simulink model "IEEE_9bus_new_wow_mach_9"  (R2013a)
settings: Solver=ode8  StartTime=0.0  StopTime=3  RelTol=1e-4
PreLoadFcn:
  | ct = 1.083
undefined symbols (not defined in the file): D1, Delta
libraries: powerlib x37, jailib x3, sps_avr x3
settings Model: Creator=jp536285  LastModifiedBy=ChakZ
settings DataIOCC: LimitDataPoints=off  SaveOutput=off  SaveTime=off
settings DebuggingCC: UnconnectedInputMsg=none  UnconnectedOutputMsg=none  UnconnectedLineMsg=none

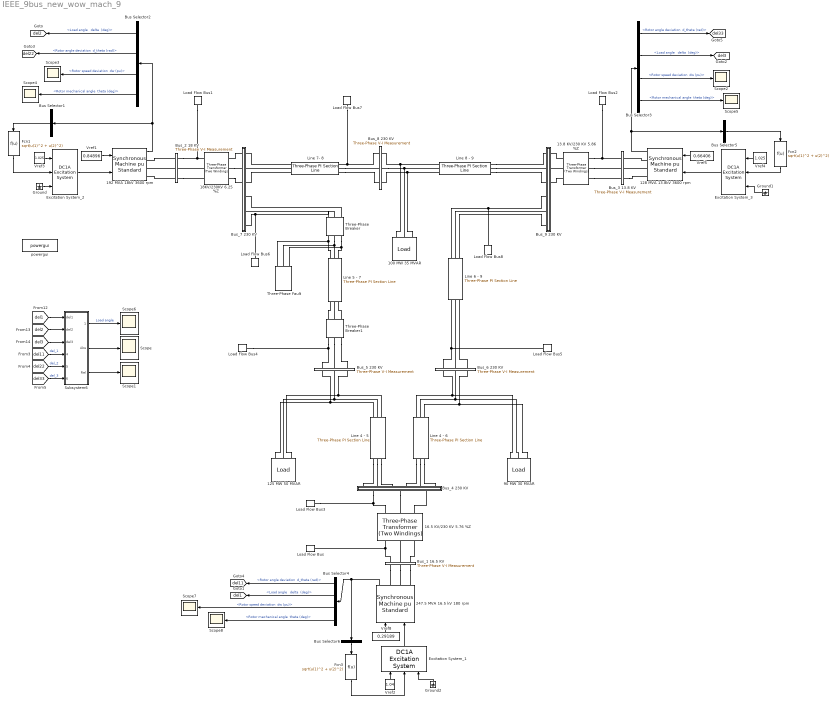
== system IEEE_9bus_new_wow_mach_9 ==
  " Line 4 - 6" : powerlib/Elements/Three-Phase PI Section Line  LConnTagsString=a|b|c  RConnTagsString=A|B|C  Frequency=60  Resistances=[ 0.08993 0.224825]  Inductances="[ 1.29e-3  3.22e-3]"  Capacitances=[7.922e-9 4.74e-9]  Length=100  mask(Three-Phase PI Section Line){}
      mask Display:
      | % This is a new mask on top of the base mask.
      | % Use "View base mask" link below to see the base mask.
      | patch([0.0 0.0 1 1 0.0 0.0 ],[0.4 0.7 0.7 0.4 0.4 0.7],[0 0 1]);
      | patch([0.4 0.4 0.42 0.42],[0.4 0.75 0.75 0.4],[1 0 0]);
      | patch([0.38 0.38 0.57 0.57],[0.7 0.75 0.75 0.7],[1 0 0]);
      | patch([0.53 0.53 0.55 0.55],[0.4 0.75 0.75 0.4],[1 0 0]);
  " Line 6 - 9" : powerlib/Elements/Three-Phase PI Section Line  LConnTagsString=a|b|c  RConnTagsString=A|B|C  Frequency=60  Resistances=[ 0.20631 0.5157]  Inductances="[ 2.38e-3  6.09e-3]"  Capacitances=[17.95e-9 10.55e-9]  Length=100  mask(Three-Phase PI Section Line){}
      mask Display:
      | % This is a new mask on top of the base mask.
      | % Use "View base mask" link below to see the base mask.
      | patch([0.0 0.0 1 1 0.0 0.0 ],[0.4 0.7 0.7 0.4 0.4 0.7],[0 0 1]);
      | patch([0.4 0.4 0.42 0.42],[0.4 0.75 0.75 0.4],[1 0 0]);
      | patch([0.38 0.38 0.57 0.57],[0.7 0.75 0.75 0.7],[1 0 0]);
      | patch([0.53 0.53 0.55 0.55],[0.4 0.75 0.75 0.4],[1 0 0]);
  100 MW 35 MVAR : jailib/Load  SystemSampleTime=-1
      link override Three-Phase Parallel RLC Load: NominalVoltage=(230000)*1.01602  ActivePower=100e6  InductivePower=35e6  LoadType=constant PQ
  125 MW 50 MVAR : jailib/Load  SystemSampleTime=-1
      link override Three-Phase Parallel RLC Load: NominalVoltage=(230000)*0.996183  ActivePower=125e6  InductivePower=50e6  LoadType=constant PQ
  128 MVA 13.8kV 3600 rpm : powerlib/Machines/Synchronous Machine pu Standard  PresetModel=No  MechanicalLoad=Mechanical power Pm  ShowDetailedParameters=on  RotorType=Round  NominalParameters="[ 128e6  13.8e3   60 ]"  Reactances1=[ 1.68, 0.23206, 0.19, 1.61, 0.23206, 0.19, 0.314]  Reactances2="[ 1.305, 0.296, 0.252, 0.474,  0.243,  0.18 ]"  dAxisTimeConstants=Open-circuit  qAxisTimeConstants=Open-circuit  TimeConstants1="[ 4.4849  0.0681  0.1  ]"  TimeConstants2=[ 5.89, 0.001,0.6, 0.001 ]  TimeConstants3="[  4.49  0.0681  0.0513  ]"  TimeConstants4=[ 8.0, 0.03, 0.3371, 0.0295 ]  TimeConstants5=[ 1.01, 0.053, 0.1 ]  TimeConstants6=[ 1.3201, 0.023, 1.0, 0.07 ]  TimeConstants7="[  1.01  0.053  0.051266  ]"  TimeConstants8=[ 1.3201, 0.0231, 0.3371, 0.0295 ]  StatorResistance=1e-7  Mechanical="[ 2.35  0 1 ]"  PolePairs=1  InitialConditions=[0 -36.0034 0.653061 0.653061 0.653061 11.785 -108.215 131.785 1.40359]  SetSaturation=off  Saturation=[0.6404,0.7127,0.8441,0.9214,0.9956,1.082,1.19,1.316,1.457;0.7,0.7698,0.8872,0.9466,0.9969,1.046,1.1,1.151,1.201]  Units=per unit standard parameters  LoadFlowParameters=[1 85000000 0 0 0]  TsPowergui=0  TsBlock=-1  IterativeModel=Trapezoidal non iterative  BusType=PV  Pref=85000000  Qref=0  Qmin=-Inf  Qmax=Inf  PLF=0  QLF=0
  13.8 KV/230 KV 5.86 %Z : powerlib/Elements/Three-Phase Transformer (Two Windings)  Winding1Connection=Delta (D1)  UNITS=pu  NominalPower=[ 100e6 , 60 ]  Winding1=[ 13.8e3 , 1e-6 , 0 ]  Winding2Connection=Yg  Winding2=[ 230e3 , 1e-6, 0.0586 ]  SetSaturation=off  Rm=500  Lm=500  Saturation=[ 0,0 ; 0.0024,1.2 ; 1.0,1.52 ]  Hysteresis=off  DataFile='hysteresis'  SetInitialFlux=off  InitialFluxes=[ 0.8 , -0.8 , 0.7 ]  Measurements=None  MoreParameters=off  BreakLoop=off  DataType=off  TransfoNumber=1
  "16.5 KV/230 KV 5.76 %Z     " : powerlib/Elements/Three-Phase Transformer (Two Windings)  Winding1Connection=Delta (D1)  UNITS=pu  NominalPower=[ 100e6 , 60 ]  Winding1=[ 16.5e3 , 1e-6, 0 ]  Winding2Connection=Yg  Winding2=[ 230e3 ,1e-6, 0.0576 ]  SetSaturation=off  Rm=500  Lm=500  Saturation=[ 0,0 ; 0.0024,1.2 ; 1.0,1.52 ]  Hysteresis=off  DataFile='hysteresis'  SetInitialFlux=off  InitialFluxes=[ 0.8 , -0.8 , 0.7 ]  Measurements=None  MoreParameters=off  BreakLoop=off  DataType=off  TransfoNumber=1
  18KV/230KV 6.25 %Z : powerlib/Elements/Three-Phase Transformer (Two Windings)  Winding1Connection=Delta (D1)  UNITS=pu  NominalPower=[ 100e6 , 60 ]  Winding1=[ 18e3 , 1e-6 , 0]  Winding2Connection=Yg  Winding2=[ 230e3 , 1e-6, 0.0625 ]  SetSaturation=off  Rm=500  Lm=500  Saturation=[ 0,0 ; 0.0024,1.2 ; 1.0,1.52 ]  Hysteresis=off  DataFile='hysteresis'  SetInitialFlux=off  InitialFluxes=[ 0.8 , -0.8 , 0.7 ]  Measurements=None  MoreParameters=off  BreakLoop=off  DataType=off  TransfoNumber=1
  192 MVA 18kV 3600 rpm : powerlib/Machines/Synchronous Machine pu Standard  PresetModel=No  MechanicalLoad=Mechanical power Pm  ShowDetailedParameters=on  RotorType=Round  NominalParameters="[ 192e6  18e3   60 ]"  Reactances1=[ 1.72, 0.23, 0.1728,1.65, 0.23, 0.1728, 0.4224 ]  Reactances2="[ 1.305, 0.296, 0.252, 0.474,  0.243,  0.18 ]"  dAxisTimeConstants=Open-circuit  qAxisTimeConstants=Open-circuit  TimeConstants1="[ 4.4849  0.0681  0.1  ]"  TimeConstants2=[ 6, 0.001, 0.53, 0.001]  TimeConstants3="[  4.49  0.0681  0.0513  ]"  TimeConstants4=[ 8.0, 0.03, 0.3371, 0.0295 ]  TimeConstants5=[ 1.01, 0.053, 0.1 ]  TimeConstants6=[ 1.3201, 0.023, 1.0, 0.07 ]  TimeConstants7="[  1.01  0.053  0.051266  ]"  TimeConstants8=[ 1.3201, 0.0231, 0.3371, 0.0295 ]  StatorResistance=1e-7  Mechanical="[ 3.33  0 1 ]"  PolePairs=1  InitialConditions=[0 -29.1799 0.828949 0.828949 0.828949 6.81655 -113.183 126.817 1.78946]  SetSaturation=off  Saturation=[0.6404,0.7127,0.8441,0.9214,0.9956,1.082,1.19,1.316,1.457;0.7,0.7698,0.8872,0.9466,0.9969,1.046,1.1,1.151,1.201]  Units=per unit standard parameters  LoadFlowParameters=[1 163000000 0 0 0]  TsPowergui=0  TsBlock=-1  IterativeModel=Trapezoidal non iterative  BusType=PV  Pref=163000000  Qref=0  Qmin=-Inf  Qmax=Inf  PLF=0  QLF=0
  247.5 MVA 16.5 kV 180 rpm : powerlib/Machines/Synchronous Machine pu Standard  PresetModel=No  MechanicalLoad=Mechanical power Pm  ShowDetailedParameters=on  RotorType=Salient-pole  NominalParameters="[ 247.5E6  16500   60 ]"  Reactances1=[ 31 32 33 34 35 36 37 ]  Reactances2=[ 0.361, 0.1504, 0.099, 0.2398, 0.099, 0.062 ]  dAxisTimeConstants=Open-circuit  qAxisTimeConstants=Open-circuit  TimeConstants1=[8.96 0.001 0.001]  TimeConstants2=[]  TimeConstants3=[]  TimeConstants4=[]  TimeConstants5=[ 1.01, 0.053, 0.31 ]  TimeConstants6=[]  TimeConstants7=[]  TimeConstants8=[]  StatorResistance=1e-7  Mechanical=[9.55 0 20]  PolePairs=20  InitialConditions=[0 -86.3839 0.299344 0.299344 0.299344 -20.3492 -140.349 99.6508 1.08182]  SetSaturation=off  Saturation=[0.6404,0.7127,0.8441,0.9214,0.9956,1.082,1.19,1.316,1.457;0.7,0.7698,0.8872,0.9466,0.9969,1.046,1.1,1.151,1.201]  Units=per unit standard parameters  LoadFlowParameters=[2 71000000 0 0]  TsPowergui=0  TsBlock=-1  IterativeModel=Trapezoidal non iterative  BusType=swing  Pref=150000000  Qref=0  Qmin=-Inf  Qmax=Inf  PLF=0  QLF=0
      settings: AttributesFormatString=\n\n
  90 MW 30 MVAR : jailib/Load  SystemSampleTime=-1
      link override Three-Phase Parallel RLC Load: NominalVoltage=(230000)*1.01315  ActivePower=90e6  InductivePower=30e6  LoadType=constant PQ
  Bus Selector1 : BusSelector  OutputSignals="dq0 components.Stator voltage  vq (pu),dq0 components.Stator voltage  vd (pu)"  OutputAsBus=on
  Bus Selector2 : BusSelector  OutputSignals="Load angle   delta  (deg),Mechanical.Rotor angle deviation  d_theta (rad),Mechanical.Rotor speed deviation  dw (pu),Mechanical.Rotor mechanical angle  theta (deg)"
  Bus Selector3 : BusSelector  OutputSignals="Mechanical.Rotor angle deviation  d_theta (rad),Load angle   delta  (deg),Mechanical.Rotor speed deviation  dw (pu),Mechanical.Rotor mechanical angle  theta (deg)"
  Bus Selector4 : BusSelector  OutputSignals="Mechanical.Rotor angle deviation  d_theta (rad),Load angle   delta  (deg),Mechanical.Rotor speed deviation  dw (pu),Mechanical.Rotor mechanical angle  theta (deg)"
  Bus Selector5 : BusSelector  OutputSignals="dq0 components.Stator voltage  vq (pu),dq0 components.Stator voltage  vd (pu)"  OutputAsBus=on
  Bus Selector6 : BusSelector  OutputSignals="dq0 components.Stator voltage  vq (pu),dq0 components.Stator voltage  vd (pu)"  OutputAsBus=on
  Bus_1 16.5 KV : powerlib/Measurements/Three-Phase V-I Measurement  VoltageMeasurement=phase-to-phase  SetLabelV=on  LabelV=Vabc_1  Vpu=on  VpuLL=off  CurrentMeasurement=yes  SetLabelI=on  LabelI=Iabc_1  Ipu=on  Pbase=100e6  Vbase=16.5e3  OutputType=Complex  PhasorSimulation=off  PSBequivalent=0
  Bus_2 18 KV : powerlib/Measurements/Three-Phase V-I Measurement  VoltageMeasurement=phase-to-phase  SetLabelV=on  LabelV=Vabc_2  Vpu=on  VpuLL=off  CurrentMeasurement=yes  SetLabelI=on  LabelI=Iabc_2  Ipu=on  Pbase=100e6  Vbase=18e3  OutputType=Complex  PhasorSimulation=off  PSBequivalent=0
  Bus_3 13.8 KV : powerlib/Measurements/Three-Phase V-I Measurement  VoltageMeasurement=phase-to-phase  SetLabelV=on  LabelV=Vabc_3  Vpu=on  VpuLL=off  CurrentMeasurement=yes  SetLabelI=on  LabelI=Iabc_3  Ipu=on  Pbase=100e6  Vbase=13.8e3  OutputType=Complex  PhasorSimulation=off  PSBequivalent=0
  Bus_4 230 KV : Subsystem
  Bus_5 230 KV : powerlib/Measurements/Three-Phase V-I Measurement  VoltageMeasurement=phase-to-ground  SetLabelV=on  LabelV=Vabc_5  Vpu=on  VpuLL=off  CurrentMeasurement=yes  SetLabelI=on  LabelI=Iabc_5  Ipu=on  Pbase=100e6  Vbase=230e3  OutputType=Complex  PhasorSimulation=off  PSBequivalent=0
  Bus_6 230 KV : powerlib/Measurements/Three-Phase V-I Measurement  VoltageMeasurement=phase-to-ground  SetLabelV=on  LabelV=Vabc_6  Vpu=on  VpuLL=off  CurrentMeasurement=yes  SetLabelI=on  LabelI=Iabc_6  Ipu=on  Pbase=100e6  Vbase=230e3  OutputType=Complex  PhasorSimulation=off  PSBequivalent=0
  Bus_7 230 KV : Subsystem
  Bus_8 230 KV : powerlib/Measurements/Three-Phase V-I Measurement  VoltageMeasurement=phase-to-ground  SetLabelV=on  LabelV=Vabc_8  Vpu=on  VpuLL=off  CurrentMeasurement=yes  SetLabelI=on  LabelI=Iabc_8  Ipu=on  Pbase=100e6  Vbase=230e3  OutputType=Complex  PhasorSimulation=off  PSBequivalent=0
  Bus_9 230 KV : Subsystem
  Excitation System_2 : sps_avr/DC1A Excitation System  Tr=20e-3  KaTa=[20 0.2]  VRminmax=[ -4 4]  KfTf=[0.063 0.35]  TbTc=[0 0]  KeTe=[1 0.314]  Efd12=[3.1 2.3]  SeEfd12=[0.483 0.1394]  v0=[1.025 1.7895]  TsBlock=0
  Excitation System_1 : sps_avr/DC1A Excitation System  Tr=20e-3  KaTa=[20 0.2]  VRminmax=[ -3 3]  KfTf=[0.063 0.35]  TbTc=[0 0]  KeTe=[1 0.314]  Efd12=[3.1 2.3]  SeEfd12=[0.483 0.1394]  v0=[1.04 1.0818]  TsBlock=0
  Excitation System_3 : sps_avr/DC1A Excitation System  Tr=20e-3  KaTa=[20 0.2]  VRminmax=[-4 4]  KfTf=[0.063 0.35]  TbTc=[0 0]  KeTe=[1 0.314]  Efd12=[3.1 2.3]  SeEfd12=[0.483 0.1394]  v0=[1.025 1.4036]  TsBlock=0
  Fcn1 : Fcn  Expr=sqrt(u(1)^2 + u(2)^2)
  Fcn2 : Fcn  Expr=sqrt(u(1)^2 + u(2)^2)
  Fcn3 : Fcn  Expr=sqrt(u(1)^2 + u(2)^2)
  Ground : Ground
  Ground1 : Ground
  Ground2 : Ground
  "Line 4 - 5 " : powerlib/Elements/Three-Phase PI Section Line  LConnTagsString=a|b|c  RConnTagsString=A|B|C  Frequency=60  Resistances=[ 0.0529 0.13225]  Inductances="[ 1.192e-3  2.38e-3]"  Capacitances=[8.82e-9 5.188e-9]  Length=100  mask(Three-Phase PI Section Line){}
      mask Display:
      | % This is a new mask on top of the base mask.
      | % Use "View base mask" link below to see the base mask.
      | patch([0.0 0.0 1 1 0.0 0.0 ],[0.4 0.7 0.7 0.4 0.4 0.7],[0 0 1]);
      | patch([0.4 0.4 0.42 0.42],[0.4 0.75 0.75 0.4],[1 0 0]);
      | patch([0.38 0.38 0.57 0.57],[0.7 0.75 0.75 0.7],[1 0 0]);
      | patch([0.53 0.53 0.55 0.55],[0.4 0.75 0.75 0.4],[1 0 0]);
  "Line 5 - 7 " : powerlib/Elements/Three-Phase PI Section Line  LConnTagsString=a|b|c  RConnTagsString=A|B|C  Frequency=60  Resistances=[ 0.16928 0.4232]  Inductances="[ 2.259e-3  5.64e-3]"  Capacitances=[15.34e-9 9.025e-9]  Length=100  mask(Three-Phase PI Section Line){}
      mask Display:
      | % This is a new mask on top of the base mask.
      | % Use "View base mask" link below to see the base mask.
      | patch([0.0 0.0 1 1 0.0 0.0 ],[0.4 0.7 0.7 0.4 0.4 0.7],[0 0 1]);
      | patch([0.4 0.4 0.42 0.42],[0.4 0.75 0.75 0.4],[1 0 0]);
      | patch([0.38 0.38 0.57 0.57],[0.7 0.75 0.75 0.7],[1 0 0]);
      | patch([0.53 0.53 0.55 0.55],[0.4 0.75 0.75 0.4],[1 0 0]);
  Line 7- 8 : powerlib/Elements/Three-Phase PI Section Line  LConnTagsString=a|b|c  RConnTagsString=A|B|C  Frequency=60  Resistances=[0.044965 0.11241]  Inductances="[ 1.01e-3  2.02e-3]"  Capacitances=[7.471e-9 4.394e-9]  Length=100  mask(Three-Phase PI Section Line){}
      mask Display:
      | % This is a new mask on top of the base mask.
      | % Use "View base mask" link below to see the base mask.
      | patch([0.0 0.0 1 1 0.0 0.0 ],[0.4 0.7 0.7 0.4 0.4 0.7],[0 0 1]);
      | patch([0.4 0.4 0.42 0.42],[0.4 0.75 0.75 0.4],[1 0 0]);
      | patch([0.38 0.38 0.57 0.57],[0.7 0.75 0.75 0.7],[1 0 0]);
      | patch([0.53 0.53 0.55 0.55],[0.4 0.75 0.75 0.4],[1 0 0]);
  Line 8 - 9 : powerlib/Elements/Three-Phase PI Section Line  LConnTagsString=a|b|c  RConnTagsString=A|B|C  Frequency=60  Resistances=[ 0.062951 0.15737]  Inductances="[ 1.414e-3  3.53e-3]"  Capacitances=[10.47e-9 6.15e-9]  Length=100  mask(Three-Phase PI Section Line){}
      mask Display:
      | % This is a new mask on top of the base mask.
      | % Use "View base mask" link below to see the base mask.
      | patch([0.0 0.0 1 1 0.0 0.0 ],[0.4 0.7 0.7 0.4 0.4 0.7],[0 0 1]);
      | patch([0.4 0.4 0.42 0.42],[0.4 0.75 0.75 0.4],[1 0 0]);
      | patch([0.38 0.38 0.57 0.57],[0.7 0.75 0.75 0.7],[1 0 0]);
      | patch([0.53 0.53 0.55 0.55],[0.4 0.75 0.75 0.4],[1 0 0]);
  Load Flow Bus : powerlib/Measurements/Load Flow Bus  LConnTagsString=a  ID=BUS_1  Vbase=16.5e3  Vref=1.04  Vangle=0  VLF=1.04  angleLF=0
      settings: AttributesFormatString=%<ID>\n%<Vbase>V\n%<VLF>pu\n%<angleLF>deg.
  Load Flow Bus1 : powerlib/Measurements/Load Flow Bus  LConnTagsString=a  ID=BUS_2  Vbase=18e3  Vref=1.025  Vangle=0  VLF=1.025  angleLF=9.166
      settings: AttributesFormatString=%<ID>\n%<Vbase>V\n%<VLF>pu\n%<angleLF>deg.
  Load Flow Bus2 : powerlib/Measurements/Load Flow Bus  LConnTagsString=a  ID=BUS_3  Vbase=13.8e3  Vref=1.025  Vangle=0  VLF=1.025  angleLF=4.553
      settings: AttributesFormatString=%<ID>\n%<Vbase>V\n%<VLF>pu\n%<angleLF>deg.
  Load Flow Bus3 : powerlib/Measurements/Load Flow Bus  LConnTagsString=a  ID=BUS_4  Vbase=230e3  Vref=1  Vangle=0  VLF=1.026  angleLF=27.77
      settings: AttributesFormatString=%<ID>\n%<Vbase>V\n%<VLF>pu\n%<angleLF>deg.
  Load Flow Bus4 : powerlib/Measurements/Load Flow Bus  LConnTagsString=a  ID=BUS_5  Vbase=230e3  Vref=1  Vangle=0  VLF=0.9962  angleLF=25.99
      settings: AttributesFormatString=%<ID>\n%<Vbase>V\n%<VLF>pu\n%<angleLF>deg.
  Load Flow Bus5 : powerlib/Measurements/Load Flow Bus  LConnTagsString=a  ID=BUS_6  Vbase=230e3  Vref=1  Vangle=0  VLF=1.013  angleLF=26.3
      settings: AttributesFormatString=%<ID>\n%<Vbase>V\n%<VLF>pu\n%<angleLF>deg.
  Load Flow Bus6 : powerlib/Measurements/Load Flow Bus  LConnTagsString=a  ID=BUS_7  Vbase=230e3  Vref=1  Vangle=0  VLF=1.026  angleLF=33.61
      settings: AttributesFormatString=%<ID>\n%<Vbase>V\n%<VLF>pu\n%<angleLF>deg.
  Load Flow Bus7 : powerlib/Measurements/Load Flow Bus  LConnTagsString=a  ID=BUS_8  Vbase=230e3  Vref=1  Vangle=0  VLF=1.016  angleLF=30.63
      settings: AttributesFormatString=%<ID>\n%<Vbase>V\n%<VLF>pu\n%<angleLF>deg.
  Load Flow Bus8 : powerlib/Measurements/Load Flow Bus  LConnTagsString=a  ID=BUS_9  Vbase=230e3  Vref=1  Vangle=0  VLF=1.032  angleLF=31.86
      settings: AttributesFormatString=%<ID>\n%<Vbase>V\n%<VLF>pu\n%<angleLF>deg.
  Scope{,1..8} (9 alike) : Scope
      Scope settings: ShowLegends=on  YMin=-100  YMax=225
      Scope1 settings: ShowLegends=on  TimeRange=3.99997  YMin=51.5  YMax=59.5
      Scope2 settings: ShowLegends=on  YMin=-7.5  YMax=12.5  SaveName=ScopeData2
      Scope3 settings: ShowLegends=on  YMin=-7.5  YMax=12.5  SaveName=ScopeData3
      Scope4 settings: ShowLegends=on  YMin=-7.5  YMax=12.5  SaveName=ScopeData4
      Scope5 settings: ShowLegends=on  YMin=-7.5  YMax=12.5  SaveName=ScopeData5
      Scope6 settings: ShowLegends=on  YMin=-200  YMax=200  SaveName=ScopeData6
      Scope7 settings: ShowLegends=on  YMin=-7.5  YMax=12.5  SaveName=ScopeData7
      Scope8 settings: ShowLegends=on  YMin=-7.5  YMax=12.5  SaveName=ScopeData8
  Subsystem6 : Subsystem
  Three-Phase Breaker : powerlib/Elements/Three-Phase Breaker  InitialState=closed  SwitchA=on  SwitchB=on  SwitchC=on  SwitchTimes=[ct]  External=off  BreakerResistance=0.001  SnubberResistance=1e7  SnubberCapacitance=inf  Measurements=None
  Three-Phase Breaker1 : powerlib/Elements/Three-Phase Breaker  InitialState=closed  SwitchA=on  SwitchB=on  SwitchC=on  SwitchTimes=[ct]  External=off  BreakerResistance=0.001  SnubberResistance=1e7  SnubberCapacitance=inf  Measurements=None
  Three-Phase Fault : powerlib/Elements/Three-Phase Fault  FaultA=on  FaultB=on  FaultC=on  FaultResistance=0.001  GroundFault=on  GroundResistance=0.001  External=off  SwitchStatus=[1 0]  SwitchTimes=[ 1 ct]  InitialStates=[0 0 1]  SnubberResistance=1e6  SnubberCapacitance=inf  Measurements=None
  Vref1 : Constant  Value=0.84896
  Vref2 : Constant  Value=1.04
  Vref3 : Constant  Value=1.025
  Vref4 : Constant  Value=1.025
  Vref5 : Constant  Value=0.66406
  Vref8 : Constant  Value=0.29189
  powergui : powerlib/powergui  Priority=1  SimulationMode=Discrete  SolverType=Backward Euler  SampleTime=5e-5  frequency=60  SPID=off  DisableSnubberDevices=off  DisableRonSwitches=off  DisableVfSwitches=off  SwTol=0  Interpol=off  DisplayEquations=off  frequencyindice=60  Pbase=10e7  ErrMax=1e-05  Iterations=50  UnitsV=kV  UnitsW=MW  FunctionMessages=off  echomessages=off  HookPort=off  EnableUseOfTLC=off  x0status=blocks  RestoreLinks=warning  ResistiveCurrentMeasurement=off  Frange=[0:2:500]  Ylog=off  Xlog=on  ShowGrid=off  save=off  variable=ZData  ZoomFFT=off  StartTime=0.0  cycles=1  DisplayStyle=1  fundamental=60  FreqAxis=off  MaxFrequency=1000  frequencyindicesteady=1  RmsSteady=1  display=off  Ts=0  methode=off
  tag scope: del11=global, del1=global, del22=global, del2=global, del33=global, del3=global
  wires:
  Vref5/1 -> 128 MVA 13.8kV 3600 rpm/1
  Excitation System_3/1 -> 128 MVA 13.8kV 3600 rpm/2
  192 MVA 18kV 3600 rpm/1 -> Bus Selector2/1, Bus Selector1/1
  Bus Selector2/1 -> [del2]  "<Load angle   delta  (deg)>"
  Bus Selector3/2 -> [del3]  "<Load angle   delta  (deg)>"
  128 MVA 13.8kV 3600 rpm/1 -> Bus Selector3/1, Bus Selector5/1
  247.5 MVA 16.5 kV 180 rpm/1 -> Bus Selector4/1, Bus Selector6/1
  Vref8/1 -> 247.5 MVA 16.5 kV 180 rpm/1
  Excitation System_1/1 -> 247.5 MVA 16.5 kV 180 rpm/2
  Bus Selector4/2 -> [del1]  "<Load angle   delta  (deg)>"
  Vref3/1 -> Excitation System_2/1
  Ground/1 -> Excitation System_2/3
  Vref4/1 -> Excitation System_3/1
  Ground1/1 -> Excitation System_3/3
  Vref2/1 -> Excitation System_1/1
  Bus Selector2/2 -> [del22]  "<Rotor angle deviation  d_theta (rad)>"
  Bus Selector4/1 -> [del11]  "<Rotor angle deviation  d_theta (rad)>"
  Bus Selector3/1 -> [del33]  "<Rotor angle deviation  d_theta (rad)>"
  Bus Selector2/3 -> Scope3/1  "<Rotor speed deviation  dw (pu)>"
  Vref1/1 -> 192 MVA 18kV 3600 rpm/1
  [del1] -> Subsystem6/1(del1)
  [del2] -> Subsystem6/2(del2)
  [del3] -> Subsystem6/3(del3)
  Subsystem6/1(Load ang) -> Scope6/1  "Load angle"
  Bus Selector2/4 -> Scope4/1  "<Rotor mechanical angle  theta (deg)>"
  Bus Selector3/3 -> Scope2/1  "<Rotor speed deviation  dw (pu)>"
  Bus Selector3/4 -> Scope5/1  "<Rotor mechanical angle  theta (deg)>"
  Bus Selector4/3 -> Scope7/1  "<Rotor speed deviation  dw (pu)>"
  Bus Selector4/4 -> Scope8/1  "<Rotor mechanical angle  theta (deg)>"
  [del11] -> Subsystem6/4(del11)  "del_1"
  [del22] -> Subsystem6/5(del22)  "del_2"
  [del33] -> Subsystem6/6(del33)  "del_3"
  Subsystem6/2(Abs) -> Scope/1
  Subsystem6/3(Rel) -> Scope1/1
  Bus Selector1/1 -> Fcn1/1
  Fcn1/1 -> Excitation System_2/2
  Excitation System_2/1 -> 192 MVA 18kV 3600 rpm/2
  Bus Selector5/1 -> Fcn2/1
  Fcn2/1 -> Excitation System_3/2
  Ground2/1 -> Excitation System_1/3
  Bus Selector6/1 -> Fcn3/1
  Fcn3/1 -> Excitation System_1/2
  connections:
  Bus_2 18 KV/LConn2 -- 192 MVA 18kV 3600 rpm/RConn2
  18KV/230KV 6.25 %Z/LConn2 -- Bus_2 18 KV/RConn2
  18KV/230KV 6.25 %Z/RConn2 -- Bus_7 230 KV/LConn2
  Bus_2 18 KV/RConn1 -- Load Flow Bus1/LConn1 -- 18KV/230KV 6.25 %Z/LConn1
  Bus_2 18 KV/RConn3 -- 18KV/230KV 6.25 %Z/LConn3
  Bus_7 230 KV/LConn1 -- 18KV/230KV 6.25 %Z/RConn1
  18KV/230KV 6.25 %Z/RConn3 -- Bus_7 230 KV/LConn3
  13.8 KV/230 KV 5.86 %Z/LConn1 -- Bus_3 13.8 KV/LConn1 -- Load Flow Bus2/LConn1
  13.8 KV/230 KV 5.86 %Z/LConn2 -- Bus_3 13.8 KV/LConn2
  13.8 KV/230 KV 5.86 %Z/LConn3 -- Bus_3 13.8 KV/LConn3
  Bus_1 16.5 KV/RConn1 -- 247.5 MVA 16.5 kV 180 rpm/RConn1
  Bus_1 16.5 KV/RConn2 -- 247.5 MVA 16.5 kV 180 rpm/RConn2
  Bus_1 16.5 KV/RConn3 -- 247.5 MVA 16.5 kV 180 rpm/RConn3
  Bus_1 16.5 KV/LConn3 -- "16.5 KV/230 KV 5.76 %Z     "/LConn3
  Bus_1 16.5 KV/LConn2 -- "16.5 KV/230 KV 5.76 %Z     "/LConn2
  13.8 KV/230 KV 5.86 %Z/RConn1 -- Bus_9 230 KV/RConn1
  13.8 KV/230 KV 5.86 %Z/RConn2 -- Bus_9 230 KV/RConn2
  13.8 KV/230 KV 5.86 %Z/RConn3 -- Bus_9 230 KV/RConn3
  Bus_4 230 KV/LConn1 -- "16.5 KV/230 KV 5.76 %Z     "/RConn1 -- Load Flow Bus3/LConn1
  Bus_4 230 KV/LConn2 -- "16.5 KV/230 KV 5.76 %Z     "/RConn2
  Line 8 - 9/LConn1 -- Bus_8 230 KV/LConn1 -- 100 MW 35 MVAR/LConn1
  Line 8 - 9/LConn2 -- 100 MW 35 MVAR/LConn2 -- Bus_8 230 KV/LConn2
  Line 8 - 9/LConn3 -- 100 MW 35 MVAR/LConn3 -- Bus_8 230 KV/LConn3
  "16.5 KV/230 KV 5.76 %Z     "/RConn3 -- Bus_4 230 KV/LConn3
  "Line 4 - 5 "/LConn1 -- 125 MW 50 MVAR/LConn1 -- Bus_5 230 KV/RConn1
  "Line 4 - 5 "/LConn2 -- 125 MW 50 MVAR/LConn2 -- Bus_5 230 KV/RConn2
  "Line 4 - 5 "/LConn3 -- 125 MW 50 MVAR/LConn3 -- Bus_5 230 KV/RConn3
  " Line 4 - 6"/LConn1 -- 90 MW 30 MVAR/LConn1 -- Bus_6 230 KV/RConn1
  " Line 4 - 6"/LConn2 -- 90 MW 30 MVAR/LConn2 -- Bus_6 230 KV/RConn2
  " Line 4 - 6"/LConn3 -- 90 MW 30 MVAR/LConn3 -- Bus_6 230 KV/RConn3
  Line 7- 8/LConn1 -- Bus_7 230 KV/RConn1
  Line 7- 8/LConn2 -- Bus_7 230 KV/RConn2
  Bus_7 230 KV/RConn3 -- Line 7- 8/LConn3
  Bus_8 230 KV/RConn1 -- Line 7- 8/RConn1 -- Load Flow Bus7/LConn1
  Line 7- 8/RConn2 -- Bus_8 230 KV/RConn2
  Line 7- 8/RConn3 -- Bus_8 230 KV/RConn3
  Line 8 - 9/RConn2 -- Bus_9 230 KV/LConn2
  Line 8 - 9/RConn1 -- Bus_9 230 KV/LConn1
  Line 8 - 9/RConn3 -- Bus_9 230 KV/LConn3
  Bus_7 230 KV/RConn6 -- Three-Phase Breaker/LConn1 -- Load Flow Bus6/LConn1
  " Line 6 - 9"/RConn1 -- Load Flow Bus8/LConn1 -- Bus_9 230 KV/LConn4
  Bus_9 230 KV/LConn5 -- " Line 6 - 9"/RConn2
  Bus_6 230 KV/LConn1 -- " Line 6 - 9"/LConn1 -- Load Flow Bus5/LConn1
  Bus_6 230 KV/LConn2 -- " Line 6 - 9"/LConn2
  Bus_6 230 KV/LConn3 -- " Line 6 - 9"/LConn3
  " Line 6 - 9"/RConn3 -- Bus_9 230 KV/LConn6
  "Line 4 - 5 "/RConn2 -- Bus_4 230 KV/RConn2
  "Line 4 - 5 "/RConn1 -- Bus_4 230 KV/RConn1
  "Line 4 - 5 "/RConn3 -- Bus_4 230 KV/RConn3
  " Line 4 - 6"/RConn2 -- Bus_4 230 KV/RConn5
  " Line 4 - 6"/RConn1 -- Bus_4 230 KV/RConn4
  " Line 4 - 6"/RConn3 -- Bus_4 230 KV/RConn6
  128 MVA 13.8kV 3600 rpm/RConn1 -- Bus_3 13.8 KV/RConn1
  128 MVA 13.8kV 3600 rpm/RConn2 -- Bus_3 13.8 KV/RConn2
  Bus_3 13.8 KV/RConn3 -- 128 MVA 13.8kV 3600 rpm/RConn3
  Bus_2 18 KV/LConn3 -- 192 MVA 18kV 3600 rpm/RConn3
  Bus_2 18 KV/LConn1 -- 192 MVA 18kV 3600 rpm/RConn1
  Bus_1 16.5 KV/LConn1 -- Load Flow Bus/LConn1 -- "16.5 KV/230 KV 5.76 %Z     "/LConn1
  Three-Phase Breaker/RConn2 -- Three-Phase Fault/LConn2 -- "Line 5 - 7 "/LConn2
  Three-Phase Breaker/RConn1 -- Three-Phase Fault/LConn1 -- "Line 5 - 7 "/LConn1
  Three-Phase Breaker/RConn3 -- Three-Phase Fault/LConn3 -- "Line 5 - 7 "/LConn3
  Three-Phase Breaker/LConn2 -- Bus_7 230 KV/RConn5
  Three-Phase Breaker/LConn3 -- Bus_7 230 KV/RConn4
  Three-Phase Breaker1/LConn2 -- "Line 5 - 7 "/RConn2
  Three-Phase Breaker1/RConn2 -- Bus_5 230 KV/LConn2
  Three-Phase Breaker1/LConn1 -- "Line 5 - 7 "/RConn1
  Three-Phase Breaker1/LConn3 -- "Line 5 - 7 "/RConn3
  Three-Phase Breaker1/RConn3 -- Bus_5 230 KV/LConn3
  Three-Phase Breaker1/RConn1 -- Load Flow Bus4/LConn1 -- Bus_5 230 KV/LConn1

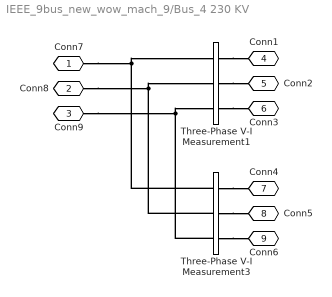
== system IEEE_9bus_new_wow_mach_9/Bus_4 230 KV ==
  Three-Phase V-I Measurement1 : powerlib/Measurements/Three-Phase V-I Measurement  VoltageMeasurement=phase-to-ground  SetLabelV=on  LabelV=Vabc_45  Vpu=on  VpuLL=off  CurrentMeasurement=yes  SetLabelI=on  LabelI=Iabc_45  Ipu=on  Pbase=100e6  Vbase=230e3  OutputType=Complex  PhasorSimulation=off  PSBequivalent=0
  Three-Phase V-I Measurement3 : powerlib/Measurements/Three-Phase V-I Measurement  VoltageMeasurement=phase-to-ground  SetLabelV=on  LabelV=Vabc_46  Vpu=on  VpuLL=off  CurrentMeasurement=yes  SetLabelI=on  LabelI=Iabc_46  Ipu=on  Pbase=100e6  Vbase=230e3  OutputType=Complex  PhasorSimulation=off  PSBequivalent=0
  Conn7 : PMIOPort  Port=1  Side=Left
  Conn8 : PMIOPort  Port=2  Side=Left
  Conn9 : PMIOPort  Port=3  Side=Left
  Conn1 : PMIOPort  Port=4  Side=Right
  Conn2 : PMIOPort  Port=5  Side=Right
  Conn3 : PMIOPort  Port=6  Side=Right
  Conn4 : PMIOPort  Port=7  Side=Right
  Conn5 : PMIOPort  Port=8  Side=Right
  Conn6 : PMIOPort  Port=9  Side=Right
  connections:
  Three-Phase V-I Measurement3/LConn3 -- Conn9/RConn1 -- Three-Phase V-I Measurement1/LConn3
  Three-Phase V-I Measurement3/LConn2 -- Conn8/RConn1 -- Three-Phase V-I Measurement1/LConn2
  Three-Phase V-I Measurement3/LConn1 -- Conn7/RConn1 -- Three-Phase V-I Measurement1/LConn1
  Three-Phase V-I Measurement3/RConn3 -- Conn6/RConn1
  Three-Phase V-I Measurement1/RConn3 -- Conn3/RConn1
  Three-Phase V-I Measurement1/RConn1 -- Conn1/RConn1
  Three-Phase V-I Measurement1/RConn2 -- Conn2/RConn1
  Three-Phase V-I Measurement3/RConn1 -- Conn4/RConn1
  Three-Phase V-I Measurement3/RConn2 -- Conn5/RConn1

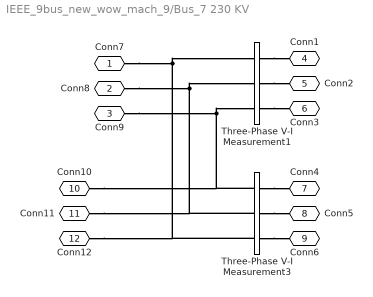
== system IEEE_9bus_new_wow_mach_9/Bus_7 230 KV ==
  Three-Phase V-I Measurement1 : powerlib/Measurements/Three-Phase V-I Measurement  VoltageMeasurement=phase-to-ground  SetLabelV=on  LabelV=Vabc_7  Vpu=on  VpuLL=off  CurrentMeasurement=yes  SetLabelI=on  LabelI=Iabc_7  Ipu=on  Pbase=100e6  Vbase=230e3  OutputType=Complex  PhasorSimulation=off  PSBequivalent=0
  Three-Phase V-I Measurement3 : powerlib/Measurements/Three-Phase V-I Measurement  VoltageMeasurement=phase-to-ground  SetLabelV=on  LabelV=Vab  Vpu=on  VpuLL=off  CurrentMeasurement=yes  SetLabelI=on  LabelI=Iab  Ipu=on  Pbase=100e6  Vbase=230e3  OutputType=Complex  PhasorSimulation=off  PSBequivalent=0
  Conn7 : PMIOPort  Port=1  Side=Left
  Conn8 : PMIOPort  Port=2  Side=Left
  Conn9 : PMIOPort  Port=3  Side=Left
  Conn1 : PMIOPort  Port=4  Side=Right
  Conn2 : PMIOPort  Port=5  Side=Right
  Conn3 : PMIOPort  Port=6  Side=Right
  Conn4 : PMIOPort  Port=7  Side=Right
  Conn5 : PMIOPort  Port=8  Side=Right
  Conn6 : PMIOPort  Port=9  Side=Right
  Conn10 : PMIOPort  Port=10  Side=Left
  Conn11 : PMIOPort  Port=11  Side=Left
  Conn12 : PMIOPort  Port=12  Side=Left
  connections:
  Three-Phase V-I Measurement3/RConn2 -- Conn5/RConn1
  Three-Phase V-I Measurement3/RConn1 -- Conn4/RConn1
  Three-Phase V-I Measurement1/RConn2 -- Conn2/RConn1
  Three-Phase V-I Measurement1/RConn1 -- Conn1/RConn1
  Three-Phase V-I Measurement1/RConn3 -- Conn3/RConn1
  Three-Phase V-I Measurement3/RConn3 -- Conn6/RConn1
  Conn7/RConn1 -- Three-Phase V-I Measurement3/LConn3 -- Conn12/RConn1 -- Three-Phase V-I Measurement1/LConn1
  Conn8/RConn1 -- Three-Phase V-I Measurement3/LConn2 -- Conn11/RConn1 -- Three-Phase V-I Measurement1/LConn2
  Conn9/RConn1 -- Conn10/RConn1 -- Three-Phase V-I Measurement3/LConn1 -- Three-Phase V-I Measurement1/LConn3

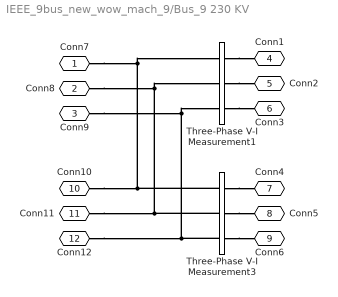
== system IEEE_9bus_new_wow_mach_9/Bus_9 230 KV ==
  Three-Phase V-I Measurement1 : powerlib/Measurements/Three-Phase V-I Measurement  VoltageMeasurement=phase-to-ground  SetLabelV=on  LabelV=Vabc_9  Vpu=on  VpuLL=off  CurrentMeasurement=yes  SetLabelI=on  LabelI=Iabc_9  Ipu=on  Pbase=100e6  Vbase=230e3  OutputType=Complex  PhasorSimulation=off  PSBequivalent=0
  Three-Phase V-I Measurement3 : powerlib/Measurements/Three-Phase V-I Measurement  VoltageMeasurement=phase-to-ground  SetLabelV=on  LabelV=Vabc  Vpu=on  VpuLL=off  CurrentMeasurement=yes  SetLabelI=on  LabelI=Iabc  Ipu=on  Pbase=100e6  Vbase=230e3  OutputType=Complex  PhasorSimulation=off  PSBequivalent=0
  Conn7 : PMIOPort  Port=1  Side=Left
  Conn8 : PMIOPort  Port=2  Side=Left
  Conn9 : PMIOPort  Port=3  Side=Left
  Conn1 : PMIOPort  Port=4  Side=Right
  Conn2 : PMIOPort  Port=5  Side=Right
  Conn3 : PMIOPort  Port=6  Side=Right
  Conn4 : PMIOPort  Port=7  Side=Right
  Conn5 : PMIOPort  Port=8  Side=Right
  Conn6 : PMIOPort  Port=9  Side=Right
  Conn10 : PMIOPort  Port=10  Side=Left
  Conn11 : PMIOPort  Port=11  Side=Left
  Conn12 : PMIOPort  Port=12  Side=Left
  connections:
  Conn12/RConn1 -- Three-Phase V-I Measurement3/LConn3 -- Conn9/RConn1 -- Three-Phase V-I Measurement1/LConn3
  Conn11/RConn1 -- Three-Phase V-I Measurement3/LConn2 -- Conn8/RConn1 -- Three-Phase V-I Measurement1/LConn2
  Conn10/RConn1 -- Three-Phase V-I Measurement3/LConn1 -- Conn7/RConn1 -- Three-Phase V-I Measurement1/LConn1
  Three-Phase V-I Measurement3/RConn3 -- Conn6/RConn1
  Three-Phase V-I Measurement1/RConn3 -- Conn3/RConn1
  Three-Phase V-I Measurement1/RConn1 -- Conn1/RConn1
  Three-Phase V-I Measurement1/RConn2 -- Conn2/RConn1
  Three-Phase V-I Measurement3/RConn1 -- Conn4/RConn1
  Three-Phase V-I Measurement3/RConn2 -- Conn5/RConn1

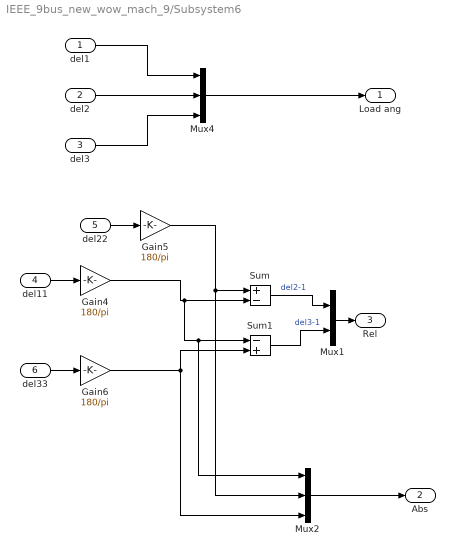
== system IEEE_9bus_new_wow_mach_9/Subsystem6 ==
  del1 : Inport
  del2 : Inport  Port=2
  del3 : Inport  Port=3
  del11 : Inport  Port=4
  del22 : Inport  Port=5
  del33 : Inport  Port=6
  Gain4 : Gain  Gain=180/pi
  Gain5 : Gain  Gain=180/pi
  Gain6 : Gain  Gain=180/pi
  Mux1 : Mux  Inputs=2
  Mux2 : Mux  Inputs=3
  Mux4 : Mux  Inputs=3
  Sum : Sum  Inputs=+-
  Sum1 : Sum  Inputs=-+
  Load ang : Outport
  Abs : Outport  Port=2
  Rel : Outport  Port=3
  wires:
  del2/1 -> Mux4/2
  Mux4/1 -> Load ang/1
  del3/1 -> Mux4/3
  del1/1 -> Mux4/1
  del11/1 -> Gain4/1
  del22/1 -> Gain5/1
  del33/1 -> Gain6/1
  Mux2/1 -> Abs/1
  Sum/1 -> Mux1/1  "del2-1"
  Sum1/1 -> Mux1/2  "del3-1"
  Mux1/1 -> Rel/1
  Gain4/1 -> Mux2/1, Sum1/1, Sum/2
  Gain5/1 -> Mux2/2, Sum/1
  Gain6/1 -> Mux2/3, Sum1/2
